simulink model "FIXED_BLOCK"  (R2024b)
settings: configuration reference "MODEL_CONFIG_CHILD" (kept outside this file)
undefined symbols (not defined in the file): BATTERY_UV_LIM_U16, BATTERY_UV_RST_LIM_U16, BOOLEAN_ONE, CONST_10000_u32, CONST_ONE_u8, CURR_CUTOFF_CTR_U16, CURRENTCUTOFF_LIM_mA_i32, DEFAULT_MAX_SPD_LIM_u16, DEFAULT_PAS_SPD_U16, DEFAULT_SPD_LIM_U16, ECO_MODE_SPD_LIM_u16, FITNESS_MODE_U8, MAX_SPD_VALUE_U16, MILLI_SEC_COUNTS_10000_U16, MILLI_SEC_COUNTS_1000_U16, MILLI_SEC_COUNTS_2000_U16, MILLI_SEC_COUNTS_3000_U16, MILLI_SEC_COUNTS_300_U16, MILLI_SEC_COUNTS_5000_U16, MIN_SPD_VALUE_U16, MOTOR_BLOCK_CTR_U16, PAS_FIVE_SPD_THSD_U16, PAS_FOUR_SPD_THSD_U16, PAS_ONE_SPD_THSD_U16, PAS_THREE_SPD_THSD_U16, PAS_TWO_SPD_THSD_U16, RPM_TO_KMPH_CONST_u32, SAMPLE_TIME_1MS, SPD_BUFFER_u16, SPD_CONV_METER_u16, SPD_PI_INIT_VAL_u16, SPD_PI_KI_u16, SPD_PI_KP_u16, THROTT_ERR_LWRTHSD_U16, THROTT_ERR_UPRTHSD_U16, THROTTLE_INITIATION_VALUE_U16, THROTTLE_SPD_LIM_U16, THROTTLE_THRESHOLD_U16, URBAN_MODE_SPD_LIM_u16, WALKMODE_SPD_LIM_U16, ZERO_i32, ZERO_U16
libraries: simulink x21, MCU_MAIN_LIB x7, slpidlib x1
settings Model: DataDictionary=MCU_FOC_MAIN_DD.sldd  EnableAccessToBaseWorkspace=off  Creator=415  LastModifiedBy=Shivaraj
settings ConfigSetRef: SourceName=MODEL_CONFIG_CHILD

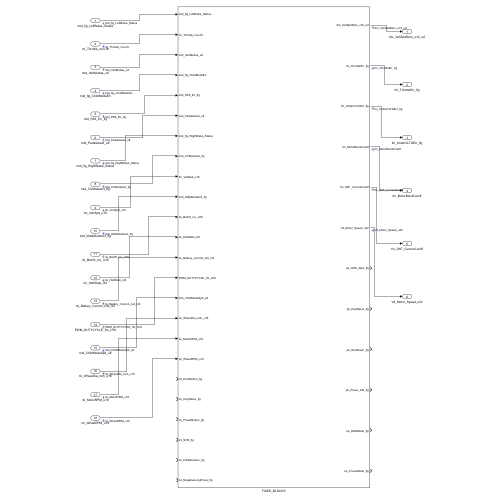
[thumbnail: Simulink's stored preview of the top-level diagram]
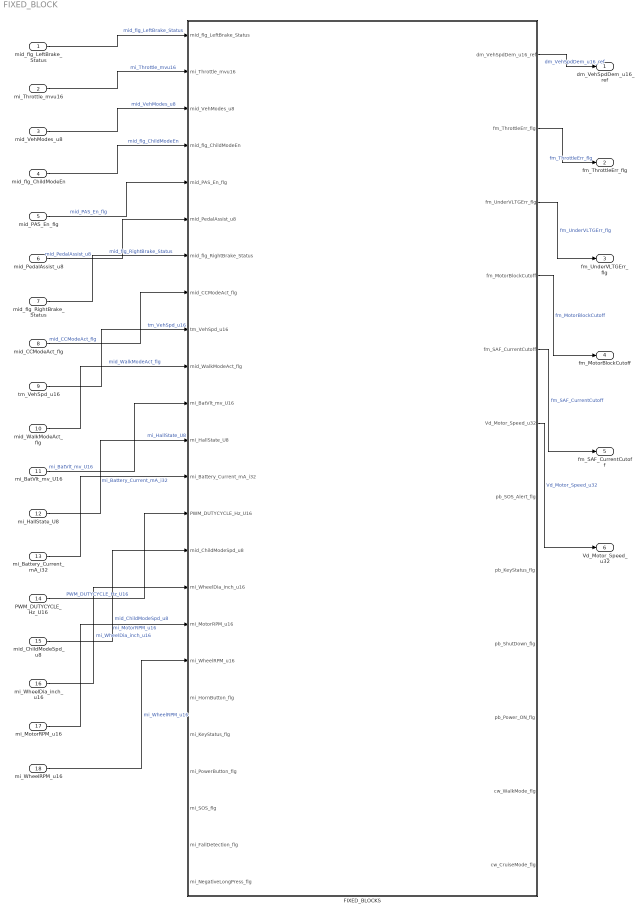
== system FIXED_BLOCK ==
  mid_flg_LeftBrake_Status : Inport
  mi_Throttle_mvu16 : Inport  Port=2
  mid_VehModes_u8 : Inport  Port=3
  mid_flg_ChildModeEn : Inport  Port=4
  mid_PAS_En_flg : Inport  Port=5
  mid_PedalAssist_u8 : Inport  Port=6
  mid_flg_RightBrake_Status : Inport  Port=7
  mid_CCModeAct_flg : Inport  Port=8
  tm_VehSpd_u16 : Inport  Port=9
  mid_WalkModeAct_flg : Inport  Port=10
  mi_BatVlt_mv_U16 : Inport  Port=11
  mi_HallState_U8 : Inport  Port=12
  mi_Battery_Current_mA_i32 : Inport  Port=13
  PWM_DUTYCYCLE_Hz_U16 : Inport  Port=14
  mid_ChildModeSpd_u8 : Inport  Port=15
  mi_WheelDia_inch_u16 : Inport  Port=16
  mi_MotorRPM_u16 : Inport  Port=17
  mi_WheelRPM_u16 : Inport  Port=18
  FIXED_BLOCKS : Subsystem
  dm_VehSpdDem_u16_ref : Outport  InitialOutput=0
  fm_ThrottleErr_flg : Outport  Port=2  InitialOutput=0
  fm_UnderVLTGErr_flg : Outport  Port=3  InitialOutput=0
  fm_MotorBlockCutoff : Outport  Port=4  InitialOutput=0
  fm_SAF_CurrentCutoff : Outport  Port=5
  Vd_Motor_Speed_u32 : Outport  Port=6  InitialOutput=0
  wires:
  FIXED_BLOCKS/4(fm_MotorBlockCutoff) -> fm_MotorBlockCutoff/1  "fm_MotorBlockCutoff"
  mid_flg_LeftBrake_Status/1 -> FIXED_BLOCKS/1(mid_flg_LeftBrake_Status)  "mid_flg_LeftBrake_Status"
  mi_Throttle_mvu16/1 -> FIXED_BLOCKS/2(mi_Throttle_mvu16)  "mi_Throttle_mvu16"
  tm_VehSpd_u16/1 -> FIXED_BLOCKS/9(tm_VehSpd_u16)  "tm_VehSpd_u16"
  mid_CCModeAct_flg/1 -> FIXED_BLOCKS/8(mid_CCModeAct_flg)  "mid_CCModeAct_flg"
  mid_ChildModeSpd_u8/1 -> FIXED_BLOCKS/15(mid_ChildModeSpd_u8)  "mid_ChildModeSpd_u8"
  mid_VehModes_u8/1 -> FIXED_BLOCKS/3(mid_VehModes_u8)  "mid_VehModes_u8"
  FIXED_BLOCKS/6(Vd_Motor_Speed_u32) -> Vd_Motor_Speed_u32/1  "Vd_Motor_Speed_u32"
  FIXED_BLOCKS/2(fm_ThrottleErr_flg) -> fm_ThrottleErr_flg/1  "fm_ThrottleErr_flg"
  mid_flg_ChildModeEn/1 -> FIXED_BLOCKS/4(mid_flg_ChildModeEn)  "mid_flg_ChildModeEn"
  mid_PAS_En_flg/1 -> FIXED_BLOCKS/5(mid_PAS_En_flg)  "mid_PAS_En_flg"
  mid_PedalAssist_u8/1 -> FIXED_BLOCKS/6(mid_PedalAssist_u8)  "mid_PedalAssist_u8"
  mid_flg_RightBrake_Status/1 -> FIXED_BLOCKS/7(mid_flg_RightBrake_Status)  "mid_flg_RightBrake_Status"
  mid_WalkModeAct_flg/1 -> FIXED_BLOCKS/10(mid_WalkModeAct_flg)  "mid_WalkModeAct_flg"
  mi_BatVlt_mv_U16/1 -> FIXED_BLOCKS/11(mi_BatVlt_mv_U16)  "mi_BatVlt_mv_U16"
  mi_HallState_U8/1 -> FIXED_BLOCKS/12(mi_HallState_U8)  "mi_HallState_U8"
  PWM_DUTYCYCLE_Hz_U16/1 -> FIXED_BLOCKS/14(PWM_DUTYCYCLE_Hz_U16)  "PWM_DUTYCYCLE_Hz_U16"
  mi_Battery_Current_mA_i32/1 -> FIXED_BLOCKS/13(mi_Battery_Current_mA_i32)  "mi_Battery_Current_mA_i32"
  mi_WheelDia_inch_u16/1 -> FIXED_BLOCKS/16(mi_WheelDia_inch_u16)  "mi_WheelDia_inch_u16"
  mi_MotorRPM_u16/1 -> FIXED_BLOCKS/17(mi_MotorRPM_u16)  "mi_MotorRPM_u16"
  mi_WheelRPM_u16/1 -> FIXED_BLOCKS/18(mi_WheelRPM_u16)  "mi_WheelRPM_u16"
  FIXED_BLOCKS/1(dm_VehSpdDem_u16_ref) -> dm_VehSpdDem_u16_ref/1  "dm_VehSpdDem_u16_ref"
  FIXED_BLOCKS/3(fm_UnderVLTGErr_flg) -> fm_UnderVLTGErr_flg/1  "fm_UnderVLTGErr_flg"
  FIXED_BLOCKS/5(fm_SAF_CurrentCutoff) -> fm_SAF_CurrentCutoff/1  "fm_SAF_CurrentCutoff"

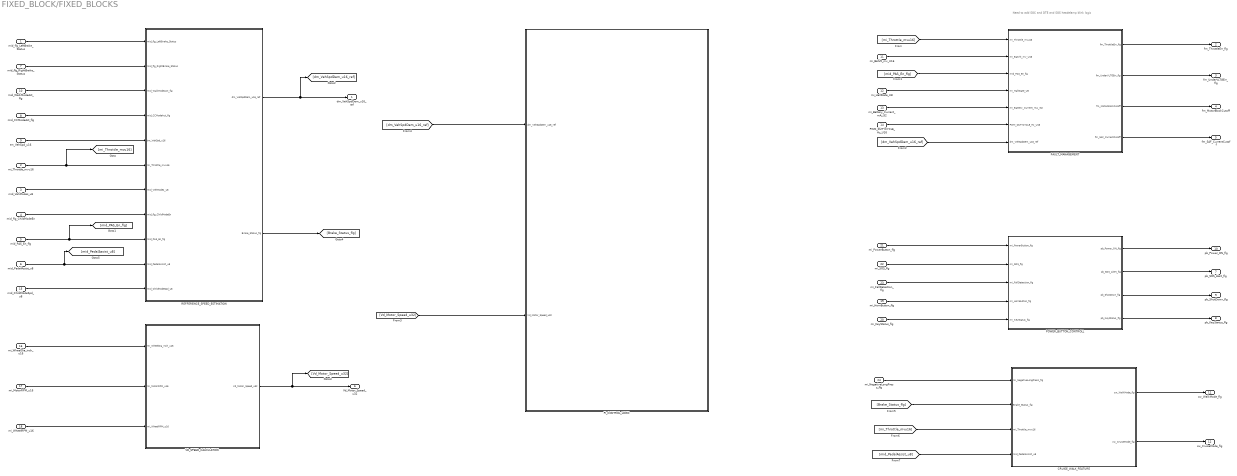
== system FIXED_BLOCK/FIXED_BLOCKS ==
  note: Need to add SOC and DTE and SOS headelamp blink logic
  mid_flg_LeftBrake_Status : Inport
  mi_Throttle_mvu16 : Inport  Port=2
  mid_VehModes_u8 : Inport  Port=3
  mid_flg_ChildModeEn : Inport  Port=4
  mid_PAS_En_flg : Inport  Port=5
  mid_PedalAssist_u8 : Inport  Port=6
  mid_flg_RightBrake_Status : Inport  Port=7
  mid_CCModeAct_flg : Inport  Port=8
  tm_VehSpd_u16 : Inport  Port=9
  mid_WalkModeAct_flg : Inport  Port=10
  mi_BatVlt_mv_U16 : Inport  Port=11
  mi_HallState_U8 : Inport  Port=12
  mi_Battery_Current_mA_i32 : Inport  Port=13
  PWM_DUTYCYCLE_Hz_U16 : Inport  Port=14
  mid_ChildModeSpd_u8 : Inport  Port=15
  mi_WheelDia_inch_u16 : Inport  Port=16
  mi_MotorRPM_u16 : Inport  Port=17
  mi_WheelRPM_u16 : Inport  Port=18
  mi_HornButton_flg : Inport  Port=19
  mi_KeyStatus_flg : Inport  Port=20
  mi_PowerButton_flg : Inport  Port=21
  mi_SOS_flg : Inport  Port=22
  mi_FallDetection_flg : Inport  Port=23
  mi_NegativeLongPress_flg : Inport  Port=24
  CRUISE_WALK_FEATURE : Subsystem
  FAULT_MANAGEMENT : Subsystem
  PI_CONTROL_LOGIC : Subsystem
  POWER_BUTTON_CONTROLL : Subsystem
  REFFERENCE_SPEED_ESTIMATION : Subsystem
  VD_SPEED_CALCULATION : Subsystem
  dm_VehSpdDem_u16_ref : Outport  InitialOutput=0
  fm_ThrottleErr_flg : Outport  Port=2
  fm_UnderVLTGErr_flg : Outport  Port=3
  fm_MotorBlockCutoff : Outport  Port=4
  fm_SAF_CurrentCutoff : Outport  Port=5
  Vd_Motor_Speed_u32 : Outport  Port=6  InitialOutput=0
  pb_SOS_Alert_flg : Outport  Port=7
  pb_KeyStatus_flg : Outport  Port=8
  pb_ShutDown_flg : Outport  Port=9
  pb_Power_ON_flg : Outport  Port=10
  cw_WalkMode_flg : Outport  Port=11
  cw_CruiseMode_flg : Outport  Port=12
  wires:
  mi_Throttle_mvu16/1 -> REFFERENCE_SPEED_ESTIMATION/6(mi_Throttle_mvu16), [mi_Throttle_mvu16]
  mid_flg_ChildModeEn/1 -> REFFERENCE_SPEED_ESTIMATION/8(mid_flg_ChildModeEn)
  mid_VehModes_u8/1 -> REFFERENCE_SPEED_ESTIMATION/7(mid_VehModes_u8)
  REFFERENCE_SPEED_ESTIMATION/1(dm_VehSpdDem_u16_ref) -> dm_VehSpdDem_u16_ref/1, [dm_VehSpdDem_u16_ref]
  mid_flg_RightBrake_Status/1 -> REFFERENCE_SPEED_ESTIMATION/2(mid_flg_RightBrake_Status)
  tm_VehSpd_u16/1 -> REFFERENCE_SPEED_ESTIMATION/5(tm_VehSpd_u16)
  mid_WalkModeAct_flg/1 -> REFFERENCE_SPEED_ESTIMATION/3(mid_WalkModeAct_flg)
  [mi_Throttle_mvu16] -> FAULT_MANAGEMENT/1(mi_Throttle_mvu16)
  mid_CCModeAct_flg/1 -> REFFERENCE_SPEED_ESTIMATION/4(mid_CCModeAct_flg)
  mid_PedalAssist_u8/1 -> [mid_PedalAssist_u8], REFFERENCE_SPEED_ESTIMATION/10(mid_PedalAssist_u8)
  mid_PAS_En_flg/1 -> [mid_PAS_En_flg], REFFERENCE_SPEED_ESTIMATION/9(mid_PAS_En_flg)
  mid_flg_LeftBrake_Status/1 -> REFFERENCE_SPEED_ESTIMATION/1(mid_flg_LeftBrake_Status)
  FAULT_MANAGEMENT/1(fm_ThrottleErr_flg) -> fm_ThrottleErr_flg/1
  mi_BatVlt_mv_U16/1 -> FAULT_MANAGEMENT/2(mi_BatVlt_mv_U16)
  [mid_PAS_En_flg] -> FAULT_MANAGEMENT/3(mid_PAS_En_flg)
  FAULT_MANAGEMENT/2(fm_UnderVLTGErr_flg) -> fm_UnderVLTGErr_flg/1
  FAULT_MANAGEMENT/3(fm_MotorBlockCutoff) -> fm_MotorBlockCutoff/1
  mi_HallState_U8/1 -> FAULT_MANAGEMENT/4(mi_HallState_U8)
  mi_Battery_Current_mA_i32/1 -> FAULT_MANAGEMENT/5(mi_Battery_Current_mA_i32)
  PWM_DUTYCYCLE_Hz_U16/1 -> FAULT_MANAGEMENT/6(PWM_DUTYCYCLE_Hz_U16)
  [dm_VehSpdDem_u16_ref] -> FAULT_MANAGEMENT/7(dm_VehSpdDem_u16_ref)
  FAULT_MANAGEMENT/4(fm_SAF_CurrentCutoff) -> fm_SAF_CurrentCutoff/1
  mid_ChildModeSpd_u8/1 -> REFFERENCE_SPEED_ESTIMATION/11(mid_ChildModeSpd_u8)
  mi_WheelDia_inch_u16/1 -> VD_SPEED_CALCULATION/1(mi_WheelDia_inch_u16)
  mi_MotorRPM_u16/1 -> VD_SPEED_CALCULATION/2(mi_MotorRPM_u16)
  mi_WheelRPM_u16/1 -> VD_SPEED_CALCULATION/3(mi_WheelRPM_u16)
  VD_SPEED_CALCULATION/1(Vd_Motor_Speed_u32) -> [Vd_Motor_Speed_u32], Vd_Motor_Speed_u32/1
  [dm_VehSpdDem_u16_ref] -> PI_CONTROL_LOGIC/1(dm_VehSpdDem_u16_ref)
  [Vd_Motor_Speed_u32] -> PI_CONTROL_LOGIC/2(Vd_Motor_Speed_u32)
  POWER_BUTTON_CONTROLL/2(pb_SOS_Alert_flg) -> pb_SOS_Alert_flg/1
  POWER_BUTTON_CONTROLL/4(pb_KeyStatus_flg) -> pb_KeyStatus_flg/1
  POWER_BUTTON_CONTROLL/3(pb_ShutDown_flg) -> pb_ShutDown_flg/1
  mi_HornButton_flg/1 -> POWER_BUTTON_CONTROLL/4(mi_HornButton_flg)
  mi_KeyStatus_flg/1 -> POWER_BUTTON_CONTROLL/5(mi_KeyStatus_flg)
  mi_FallDetection_flg/1 -> POWER_BUTTON_CONTROLL/3(mi_FallDetection_flg)
  mi_SOS_flg/1 -> POWER_BUTTON_CONTROLL/2(mi_SOS_flg)
  mi_PowerButton_flg/1 -> POWER_BUTTON_CONTROLL/1(mi_PowerButton_flg)
  POWER_BUTTON_CONTROLL/1(pb_Power_ON_flg) -> pb_Power_ON_flg/1
  REFFERENCE_SPEED_ESTIMATION/2(Brake_Status_flg) -> [Brake_Status_flg]
  [Brake_Status_flg] -> CRUISE_WALK_FEATURE/2(Brake_Status_flg)
  [mi_Throttle_mvu16] -> CRUISE_WALK_FEATURE/3(mi_Throttle_mvu16)
  [mid_PedalAssist_u8] -> CRUISE_WALK_FEATURE/4(mid_PedalAssist_u8)
  CRUISE_WALK_FEATURE/1(cw_WalkMode_flg) -> cw_WalkMode_flg/1
  CRUISE_WALK_FEATURE/2(cw_CruiseMode_flg) -> cw_CruiseMode_flg/1
  mi_NegativeLongPress_flg/1 -> CRUISE_WALK_FEATURE/1(mi_NegativeLongPress_flg)

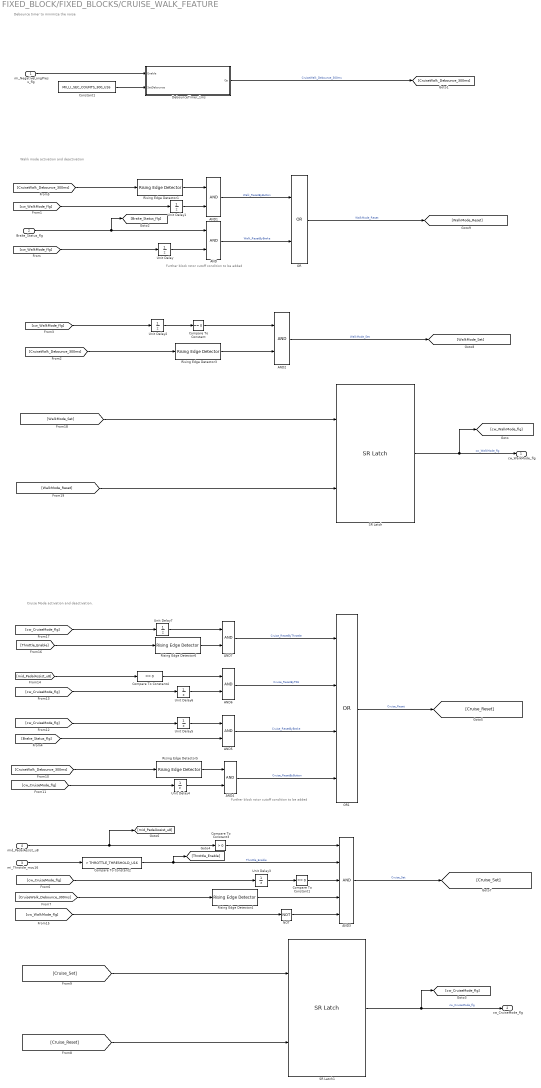
== system FIXED_BLOCK/FIXED_BLOCKS/CRUISE_WALK_FEATURE ==
  note: Debounce timer to minimize the noise
  note: Cruise Mode activation and deactivation.
  note: Walik mode activation and deactivation
  note: Further block rotor cutoff condition to be added
  note: Further block rotor cutoff condition to be added
  mi_NegativeLongPress_flg : Inport
  Brake_Status_flg : Inport  Port=2
  mi_Throttle_mvu16 : Inport  Port=3
  mid_PedalAssist_u8 : Inport  Port=4
  AND{,1..2,4..7} (7 alike) : Logic  AllPortsSameDT=off  OutDataTypeStr=boolean
  AND3 : Logic  Inputs=5  AllPortsSameDT=off  OutDataTypeStr=boolean
  Compare To Constant : simulink/Logic and Bit Operations/Compare To Constant  relop===  const=0  OutDataTypeStr=boolean
  Compare To Constant1 : simulink/Logic and Bit Operations/Compare To Constant  relop===  const=0  OutDataTypeStr=boolean
  Compare To Constant2 : simulink/Logic and Bit Operations/Compare To Constant  relop=>  const=THROTTLE_THRESHOLD_U16  OutDataTypeStr=boolean
  Compare To Constant3 : simulink/Logic and Bit Operations/Compare To Constant  relop=>  const=0  OutDataTypeStr=boolean
  Compare To Constant4 : simulink/Logic and Bit Operations/Compare To Constant  relop===  const=0  OutDataTypeStr=boolean
  Constant1 : Constant  Value=MILLI_SEC_COUNTS_300_U16
  DebounceTimer_1ms : Subsystem
  NOT : Logic  Operator=NOT  IconShape=distinctive  AllPortsSameDT=off  OutDataTypeStr=boolean
  OR : Logic  Operator=OR  AllPortsSameDT=off  OutDataTypeStr=boolean
  OR1 : Logic  Operator=OR  Inputs=4  AllPortsSameDT=off  OutDataTypeStr=boolean
  Rising Edge Detector{1,3..6} (5 alike) : MCU_MAIN_LIB/Rising Edge Detector  SystemSampleTime=-1  VariantActivationTime=update diagram  AllowFlexibleInterface=on  Latency=0  AutoFrameSizeCalculation=off
  SR Latch : MCU_MAIN_LIB/SR Latch  SystemSampleTime=-1  VariantActivationTime=update diagram  AllowFlexibleInterface=on  Latency=0  AutoFrameSizeCalculation=off
  SR Latch1 : MCU_MAIN_LIB/SR Latch  SystemSampleTime=-1  VariantActivationTime=update diagram  AllowFlexibleInterface=on  Latency=0  AutoFrameSizeCalculation=off
  Unit Delay{,1..7} (8 alike) : UnitDelay  SampleTime=-1  HasFrameUpgradeWarning=on
  cw_WalkMode_flg : Outport
  cw_CruiseMode_flg : Outport  Port=2
  wires:
  mi_NegativeLongPress_flg/1 -> DebounceTimer_1ms/1(Enable)
  Constant1/1 -> DebounceTimer_1ms/2(SetDebounce)
  SR Latch/1 -> [cw_WalkMode_flg], cw_WalkMode_flg/1  "cw_WalkMode_flg"
  AND/1 -> OR/2  "Walk_ResetByBrake"
  [cw_WalkMode_flg] -> Unit Delay/1
  Unit Delay/1 -> AND/2
  Brake_Status_flg/1 -> [Brake_Status_flg], AND/1
  Unit Delay1/1 -> AND1/2
  [cw_WalkMode_flg] -> Unit Delay1/1
  AND1/1 -> OR/1  "Walk_ResetByButton"
  Rising Edge Detector1/1 -> AND1/1
  [CruiseWalk_Debounce_300ms] -> Rising Edge Detector1/1
  DebounceTimer_1ms/1(Op) -> [CruiseWalk_Debounce_300ms]  "CruiseWalk_Debounce_300ms"
  [cw_WalkMode_flg] -> Unit Delay2/1
  Unit Delay2/1 -> Compare To Constant/1
  Compare To Constant/1 -> AND2/1
  SR Latch1/1 -> [cw_CruiseMode_flg], cw_CruiseMode_flg/1  "cw_CruiseMode_flg"
  Unit Delay3/1 -> Compare To Constant1/1
  [cw_CruiseMode_flg] -> Unit Delay3/1
  mi_Throttle_mvu16/1 -> Compare To Constant2/1
  Compare To Constant1/1 -> AND3/3
  [CruiseWalk_Debounce_300ms] -> Rising Edge Detector4/1
  Compare To Constant2/1 -> [Throttle_Enable], AND3/2  "Throttle_Enable"
  Compare To Constant3/1 -> AND3/1
  mid_PedalAssist_u8/1 -> [mid_PedalAssist_u8], Compare To Constant3/1
  Rising Edge Detector3/1 -> AND2/2
  Rising Edge Detector4/1 -> AND3/4
  [CruiseWalk_Debounce_300ms] -> Rising Edge Detector5/1
  Rising Edge Detector5/1 -> AND4/1
  [cw_CruiseMode_flg] -> Unit Delay4/1
  Unit Delay4/1 -> AND4/2
  Unit Delay5/1 -> AND5/1
  [cw_CruiseMode_flg] -> Unit Delay5/1
  Unit Delay6/1 -> AND6/2
  [cw_CruiseMode_flg] -> Unit Delay6/1
  [mid_PedalAssist_u8] -> Compare To Constant4/1
  Compare To Constant4/1 -> AND6/1
  [cw_WalkMode_flg] -> NOT/1
  NOT/1 -> AND3/5
  Rising Edge Detector6/1 -> AND7/2
  [Throttle_Enable] -> Rising Edge Detector6/1
  [cw_CruiseMode_flg] -> Unit Delay7/1
  Unit Delay7/1 -> AND7/1
  [CruiseWalk_Debounce_300ms] -> Rising Edge Detector3/1
  AND4/1 -> OR1/4  "Cruise_ResetByButton"
  [Brake_Status_flg] -> AND5/2
  AND7/1 -> OR1/1  "Cruise_ResetByThrottle"
  AND6/1 -> OR1/2  "Cruise_ResetByPAS"
  AND5/1 -> OR1/3  "Cruise_ResetByBrake"
  OR1/1 -> [Cruise_Reset]  "Cruise_Reset"
  [Cruise_Reset] -> SR Latch1/2
  AND3/1 -> [Cruise_Set]  "Cruise_Set"
  [Cruise_Set] -> SR Latch1/1
  AND2/1 -> [WalkMode_Set]  "WalkMode_Set"
  [WalkMode_Set] -> SR Latch/1
  OR/1 -> [WalkMode_Reset]  "WalkMode_Reset"
  [WalkMode_Reset] -> SR Latch/2

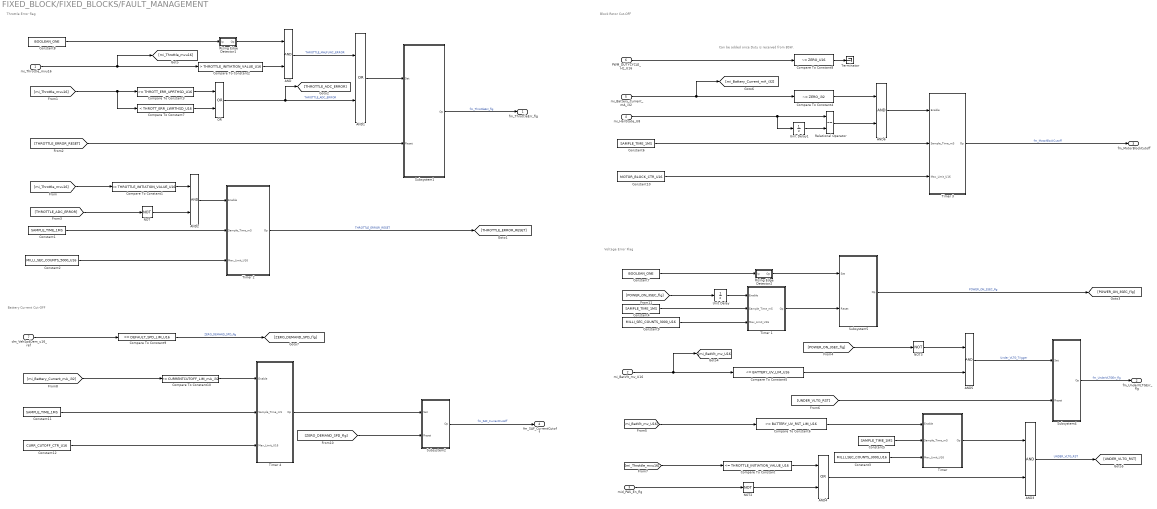
== system FIXED_BLOCK/FIXED_BLOCKS/FAULT_MANAGEMENT ==
  note: Battery Current Cut-OFF
  note: Can be added once Duty is received from BSW.
  note: Block Rotor Cut-OFF
  note: Voltage Error Flag
  note: Throttle Error flag
  mi_Throttle_mvu16 : Inport
  mi_BatVlt_mv_U16 : Inport  Port=2
  mid_PAS_En_flg : Inport  Port=3
  mi_HallState_U8 : Inport  Port=4
  mi_Battery_Current_mA_i32 : Inport  Port=5
  PWM_DUTYCYCLE_Hz_U16 : Inport  Port=6
  dm_VehSpdDem_u16_ref : Inport  Port=7
  AND{,2..3,5..6} (5 alike) : Logic  AllPortsSameDT=off  OutDataTypeStr=boolean
  AND1 : Logic  Operator=OR  AllPortsSameDT=off  OutDataTypeStr=boolean
  AND4 : Logic  Operator=OR  AllPortsSameDT=off  OutDataTypeStr=boolean
  Compare To Constant : simulink/Logic and Bit Operations/Compare To Constant  relop=<=  const=THROTTLE_INITIATION_VALUE_U16  OutDataTypeStr=boolean
  Compare To Constant1 : simulink/Logic and Bit Operations/Compare To Constant  relop=<=  const=THROTTLE_INITIATION_VALUE_U16  OutDataTypeStr=boolean
  Compare To Constant10 : simulink/Logic and Bit Operations/Compare To Constant  relop=>=  const=CURRENTCUTOFF_LIM_mA_i32  OutDataTypeStr=boolean
  Compare To Constant2 : simulink/Logic and Bit Operations/Compare To Constant  relop=>  const=THROTTLE_INITIATION_VALUE_U16  OutDataTypeStr=boolean
  Compare To Constant3 : simulink/Logic and Bit Operations/Compare To Constant  relop=>=  const=THROTT_ERR_UPRTHSD_U16  OutDataTypeStr=boolean
  Compare To Constant4 : simulink/Logic and Bit Operations/Compare To Constant  relop=~=  const=ZERO_i32  OutDataTypeStr=boolean
  Compare To Constant5 : simulink/Logic and Bit Operations/Compare To Constant  relop=<=  const=BATTERY_UV_LIM_U16  OutDataTypeStr=boolean
  Compare To Constant6 : simulink/Logic and Bit Operations/Compare To Constant  relop=>=  const=BATTERY_UV_RST_LIM_U16  OutDataTypeStr=boolean
  Compare To Constant7 : simulink/Logic and Bit Operations/Compare To Constant  relop=<  const=THROTT_ERR_LWRTHSD_U16  OutDataTypeStr=boolean
  Compare To Constant8 : simulink/Logic and Bit Operations/Compare To Constant  relop=~=  const=ZERO_U16  OutDataTypeStr=boolean
  Compare To Constant9 : simulink/Logic and Bit Operations/Compare To Constant  relop===  const=DEFAULT_SPD_LIM_U16  OutDataTypeStr=boolean
  Constant{1,4..6,11} (5 alike) : Constant  Value=SAMPLE_TIME_1MS
  Constant10 : Constant  Value=MOTOR_BLOCK_CTR_U16
  Constant12 : Constant  Value=CURR_CUTOFF_CTR_U16
  Constant2 : Constant  Value=MILLI_SEC_COUNTS_5000_U16
  Constant3 : Constant  Value=MILLI_SEC_COUNTS_3000_U16
  Constant7 : Constant  Value=BOOLEAN_ONE
  Constant8 : Constant  Value=BOOLEAN_ONE
  Constant9 : Constant  Value=MILLI_SEC_COUNTS_3000_U16
  NOT : Logic  Operator=NOT  IconShape=distinctive  AllPortsSameDT=off  OutDataTypeStr=boolean
  NOT2 : Logic  Operator=NOT  IconShape=distinctive  AllPortsSameDT=off  OutDataTypeStr=boolean
  NOT3 : Logic  Operator=NOT  IconShape=distinctive  AllPortsSameDT=off  OutDataTypeStr=boolean
  OR : Logic  Operator=OR  AllPortsSameDT=off  OutDataTypeStr=boolean
  Relational Operator : RelationalOperator  Operator===  OutDataTypeStr=boolean  RndMeth=Simplest  InputSameDT=off
  Rising Edge Detector1 : Subsystem
  Rising Edge Detector2 : Subsystem
  Subsystem1 : Subsystem
  Subsystem2 : Subsystem
  Subsystem4 : Subsystem
  Subsystem5 : Subsystem
  Terminator : Terminator
  "Timer " : Subsystem
  Timer 1 : Subsystem
  Timer 2 : Subsystem
  Timer 3 : Subsystem
  Timer 4 : Subsystem
  Unit Delay : UnitDelay  SampleTime=-1  HasFrameUpgradeWarning=on
  Unit Delay1 : UnitDelay  SampleTime=-1  HasFrameUpgradeWarning=on
  fm_ThrottleErr_flg : Outport
  fm_UnderVLTGErr_flg : Outport  Port=2
  fm_MotorBlockCutoff : Outport  Port=3  OutputWhenDisabled=reset  InitialOutput=0
  fm_SAF_CurrentCutoff : Outport  Port=4  OutputWhenDisabled=reset  InitialOutput=0
  wires:
  Constant8/1 -> Rising Edge Detector1/1(Ip)
  mi_Throttle_mvu16/1 -> Compare To Constant2/1, [mi_Throttle_mvu16]
  Compare To Constant2/1 -> AND/2
  Rising Edge Detector1/1(Op) -> AND/1
  AND/1 -> AND1/1  "THROTTLE_MALFUNC_ERROR"
  Timer 2/1(Op) -> [THROTTLE_ERROR_RESET]  "THROTTLE_ERROR_RESET"
  Constant1/1 -> Timer 2/2(Sample_Time_mS)
  Compare To Constant1/1 -> AND2/1
  [mi_Throttle_mvu16] -> Compare To Constant1/1
  Constant2/1 -> Timer 2/3(Max_Limit_U16)
  Subsystem1/1(Op) -> fm_ThrottleErr_flg/1  "fm_ThrottleErr_flg"
  Compare To Constant7/1 -> OR/2
  Compare To Constant3/1 -> OR/1
  [THROTTLE_ERROR_RESET] -> Subsystem1/2(Reset)
  AND1/1 -> Subsystem1/1(Set)
  [mi_Throttle_mvu16] -> Compare To Constant3/1, Compare To Constant7/1
  OR/1 -> [THROTTLE_ADC_ERROR], AND1/2  "THROTTLE_ADC_ERROR"
  [THROTTLE_ADC_ERROR] -> NOT/1
  NOT/1 -> AND2/2
  AND2/1 -> Timer 2/1(Enable)
  Unit Delay/1 -> Timer 1/1(Enable)
  NOT3/1 -> AND5/1
  NOT2/1 -> AND4/2
  Subsystem5/1(Op) -> [POWER_ON_3SEC_flg]  "POWER_ON_3SEC_flg"
  Subsystem4/1(Op) -> fm_UnderVLTGErr_flg/1  "fm_UnderVLTGErr_flg"
  Compare To Constant5/1 -> AND5/2
  mid_PAS_En_flg/1 -> NOT2/1
  [mi_Throttle_mvu16] -> Compare To Constant/1
  Constant9/1 -> Timer 1/3(Max_Limit_U16)
  Constant4/1 -> Timer 1/2(Sample_Time_mS)
  Constant5/1 -> "Timer "/2(Sample_Time_mS)
  Rising Edge Detector2/1(Op) -> Subsystem5/1(Set)
  Compare To Constant6/1 -> "Timer "/1(Enable)
  Compare To Constant/1 -> AND4/1
  [POWER_ON_3SEC_flg] -> Unit Delay/1
  Constant7/1 -> Rising Edge Detector2/1(Ip)
  AND5/1 -> Subsystem4/1(Set)  "Under_VLTG_Trigger"
  mi_BatVlt_mv_U16/1 -> [mi_BatVlt_mv_U16], Compare To Constant5/1
  "Timer "/1(Op) -> AND3/1
  AND4/1 -> AND3/2
  Timer 1/1(Op) -> Subsystem5/2(Reset)
  [UNDER_VLTG_RST] -> Subsystem4/2(Reset)
  Constant3/1 -> "Timer "/3(Max_Limit_U16)
  [POWER_ON_3SEC_flg] -> NOT3/1
  [mi_BatVlt_mv_U16] -> Compare To Constant6/1
  AND3/1 -> [UNDER_VLTG_RST]  "UNDER_VLTG_RST"
  Timer 3/1(Op) -> fm_MotorBlockCutoff/1  "fm_MotorBlockCutoff"
  AND6/1 -> Timer 3/1(Enable)
  Relational Operator/1 -> AND6/2
  Compare To Constant4/1 -> AND6/1
  mi_Battery_Current_mA_i32/1 -> Compare To Constant4/1, [mi_Battery_Current_mA_i32]
  Unit Delay1/1 -> Relational Operator/2
  mi_HallState_U8/1 -> Unit Delay1/1, Relational Operator/1
  Constant6/1 -> Timer 3/2(Sample_Time_mS)
  Constant10/1 -> Timer 3/3(Max_Limit_U16)
  Compare To Constant8/1 -> Terminator/1
  PWM_DUTYCYCLE_Hz_U16/1 -> Compare To Constant8/1
  Constant11/1 -> Timer 4/2(Sample_Time_mS)
  Compare To Constant10/1 -> Timer 4/1(Enable)
  [mi_Battery_Current_mA_i32] -> Compare To Constant10/1
  Timer 4/1(Op) -> Subsystem2/1(Set)
  Constant12/1 -> Timer 4/3(Max_Limit_U16)
  dm_VehSpdDem_u16_ref/1 -> Compare To Constant9/1
  Compare To Constant9/1 -> [ZERO_DEMAND_SPD_flg]  "ZERO_DEMAND_SPD_flg"
  [ZERO_DEMAND_SPD_flg] -> Subsystem2/2(Reset)
  Subsystem2/1(Op) -> fm_SAF_CurrentCutoff/1  "fm_SAF_CurrentCutoff"

== system FIXED_BLOCK/FIXED_BLOCKS/PI_CONTROL_LOGIC ==
  dm_VehSpdDem_u16_ref : Inport
  Vd_Motor_Speed_u32 : Inport  Port=2
  Add : Sum  Inputs=+-
  Constant : Constant  Value=SPD_PI_KP_u16
  Constant1 : Constant  Value=SPD_PI_KI_u16
  Constant2 : Constant  Value=SPD_PI_INIT_VAL_u16
  PID Controller : slpidlib/PID Controller  Controller=PI  Form=Parallel  TimeDomain=Discrete-time  UseExternalTs=off  SampleTime=-1  IntegratorMethod=Forward Euler  FilterMethod=Forward Euler  ControllerParametersSource=external  P=1  I=1  UseKiTs=on  D=0  UseExternalDerivativeSource=off  N=100  UseFilter=on  TunerSelectOption=Transfer Function Based (PID Tuner App)  InitialConditionSource=external  InitialConditionForIntegrator=0  InitialConditionForFilter=0  DifferentiatorICPrevScaledInput=0  ExternalReset=none  TrackingMode=off  Kt=1  LimitOutput=on  SatLimitsSource=external  UpperSaturationLimit=inf  LowerSaturationLimit=-inf  LinearizeAsGain=on  AntiWindupMode=none  Kb=1  LimitIntegrator=off  UpperIntegratorSaturationLimit=inf  LowerIntegratorSaturationLimit=-inf  SaturateOnIntegerOverflow=on  PGainOutDataTypeStr=Inherit: Inherit via back propagation  PProdOutDataTypeStr=Inherit: Inherit via back propagation  POutMin=[]  POutMax=[]  IGainOutDataTypeStr=Inherit: Inherit via back propagation  IProdOutDataTypeStr=Inherit: Inherit via back propagation  IOutMin=[]  IOutMax=[]  DOutMin=[]  DOutMax=[]  NOutMin=[]  NOutMax=[]  SumOutDataTypeStr=Inherit: Inherit via back propagation  SumOutMin=[]  SumOutMax=[]  SaturationOutMin=[]  SaturationOutMax=[]  PParamMin=[]  PParamMax=[]  IParamMin=[]  IParamMax=[]  DParamMin=[]  DParamMax=[]  NParamMin=[]  NParamMax=[]  KbParamMin=[]  KbParamMax=[]  KtParamMin=[]  KtParamMax=[]  KbOutMin=[]  KbOutMax=[]  KtOutMin=[]  KtOutMax=[]  IntegratorOutDataTypeStr=Inherit: Inherit via back propagation  IntegratorOutMin=[]  IntegratorOutMax=[]  FilterOutMin=[]  FilterOutMax=[]  SumI1OutMin=[]  SumI1OutMax=[]  SumI2OutMin=[]  SumI2OutMax=[]  SumI3OutMin=[]  SumI3OutMax=[]  SumI4OutMin=[]  SumI4OutMax=[]  SumDOutMin=[]  SumDOutMax=[]  DifferentiatorOutMin=[]  DifferentiatorOutMax=[]  FilterDiffOutCoefMin=[]  FilterDiffOutCoefMax=[]  ReciprocalOutMin=[]  ReciprocalOutMax=[]  SumDenOutMin=[]  SumDenOutMax=[]  SumNumOutMin=[]  SumNumOutMax=[]  DivideOutMin=[]  DivideOutMax=[]  UdiffTsProdOutMin=[]  UdiffTsProdOutMax=[]  NTsProdOutMin=[]  NTsProdOutMax=[]  UintegralTsProdOutMin=[]  UintegralTsProdOutMax=[]  UngainTsProdOutMin=[]  UngainTsProdOutMax=[]  ClampingZeroOutDataTypeStr=Inherit: Inherit via back propagation  ClampingZeroOutMin=[]  ClampingZeroOutMax=[]  FilterDenConstantOutDataTypeStr=Inherit: Inherit via back propagation  FilterDenConstantOutMin=[]  FilterDenConstantOutMax=[]  PCopyOutDataTypeStr=Inherit: Inherit via back propagation  PCopyOutMin=[]  PCopyOutMax=[]  NCopyOutDataTypeStr=Inherit: Inherit via back propagation  NCopyOutMin=[]  NCopyOutMax=[]  IntegratorContinuousStateAttributes=''  IntegratorStateMustResolveToSignalObject=off  IntegratorRTWStateStorageClass=Auto  FilterContinuousStateAttributes=''  FilterStateMustResolveToSignalObject=off  FilterRTWStateStorageClass=Auto  ParallelPVariant=ExternalParameters  IdealPVariant=Disabled  IVariant=ExternalParameters  DVariant=Disabled  IntegratorVariant=Discrete  SatVariant=External  AWVariant=Passthrough  PCopyVariant=Disabled  TRVariant=Disabled  FdbkBlocksVariant=Forward  IdealPFdbkVariant=Disabled  SatFdbkVariant=Disabled  DerivativeFilterVariant=Disabled  NVariant=Disabled  NCopyVariant=Disabled_SignalSpec  FilterICVariant=Disabled  IntegratorICVariant=ExternalICs  ExternalResetVariant=Disabled  TRSumVariant=Passthrough  SumFdbkVariant=Disabled  SumVariant=Sum_PI  TsampFilterVariant=InternalTs  TsampNgainVariant=Passthrough  TsampIntegralVariant=Disabled_SignalSpec  ExternalSaturationOutDataTypeStr=Inherit: Same as second input  DerivativeSourceVariant=Disabled  PreIntVariant=InternalPreInt
  wires:
  Constant2/1 -> PID Controller/4
  Constant1/1 -> PID Controller/3
  Constant/1 -> PID Controller/2
  Vd_Motor_Speed_u32/1 -> Add/2
  dm_VehSpdDem_u16_ref/1 -> Add/1
  Add/1 -> PID Controller/1

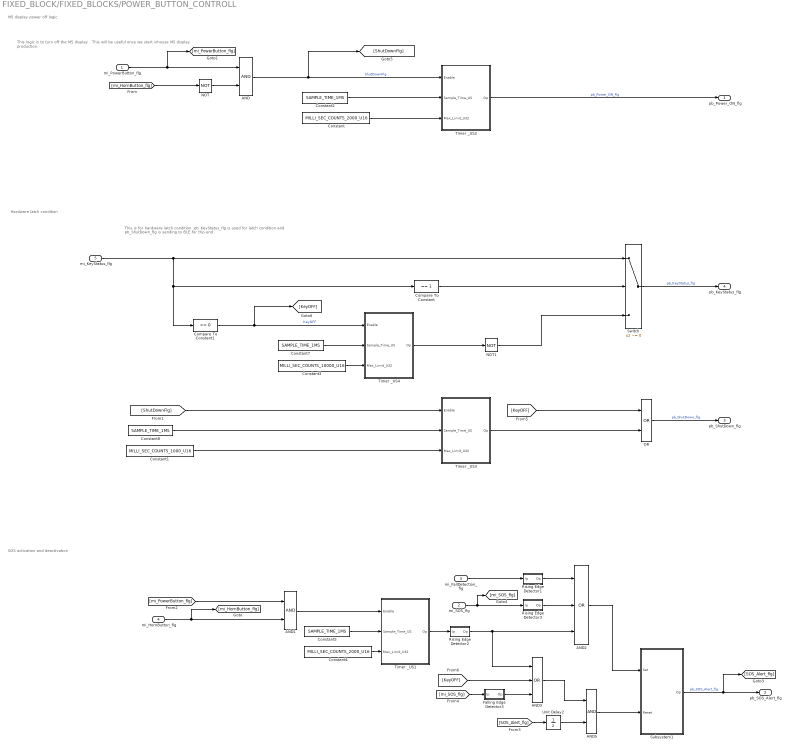
== system FIXED_BLOCK/FIXED_BLOCKS/POWER_BUTTON_CONTROLL ==
  note: This logic is to turn off the M5 display . This will be useful once we start inhouse M5 display production.
  note: M5 display power off logic
  note: This is for hardware latch condition .pb_KeyStatus_flg is used for latch condition and pb_ShutDown_flg is sending to BLE for trip end .
  note: Hardware latch condition
  note: SOS activation and deactivation
  mi_PowerButton_flg : Inport
  mi_SOS_flg : Inport  Port=2
  mi_FallDetection_flg : Inport  Port=3
  mi_HornButton_flg : Inport  Port=4
  mi_KeyStatus_flg : Inport  Port=5
  AND : Logic  AllPortsSameDT=off  OutDataTypeStr=boolean
  AND1 : Logic  AllPortsSameDT=off  OutDataTypeStr=boolean
  AND2 : Logic  Operator=OR  Inputs=3  AllPortsSameDT=off  OutDataTypeStr=boolean
  AND3 : Logic  Operator=OR  Inputs=3  AllPortsSameDT=off  OutDataTypeStr=boolean
  AND5 : Logic  AllPortsSameDT=off  OutDataTypeStr=boolean
  Compare To Constant : simulink/Logic and Bit Operations/Compare To Constant  relop===  const=1  OutDataTypeStr=boolean
  Compare To Constant1 : simulink/Logic and Bit Operations/Compare To Constant  relop===  const=0  OutDataTypeStr=boolean
  Constant : Constant  Value=MILLI_SEC_COUNTS_2000_U16
  Constant1 : Constant  Value=MILLI_SEC_COUNTS_1000_U16
  Constant{2,5,7..8} (4 alike) : Constant  Value=SAMPLE_TIME_1MS
  Constant3 : Constant  Value=MILLI_SEC_COUNTS_10000_U16
  Constant4 : Constant  Value=MILLI_SEC_COUNTS_2000_U16
  Falling Edge Detector3 : Subsystem
  NOT : Logic  Operator=NOT  AllPortsSameDT=off  OutDataTypeStr=boolean
  NOT1 : Logic  Operator=NOT  IconShape=distinctive  AllPortsSameDT=off  OutDataTypeStr=boolean
  OR : Logic  Operator=OR  AllPortsSameDT=off  OutDataTypeStr=boolean
  Rising Edge Detector1 : Subsystem
  Rising Edge Detector2 : Subsystem
  Rising Edge Detector3 : Subsystem
  Subsystem1 : Subsystem
  Switch : Switch  Criteria=u2 ~= 0  SaturateOnIntegerOverflow=off  InputSameDT=off
  Timer _US1 : Subsystem
  Timer _US2 : Subsystem
  Timer _US3 : Subsystem
  Timer _US4 : Subsystem
  Unit Delay2 : UnitDelay  SampleTime=-1  HasFrameUpgradeWarning=on
  pb_Power_ON_flg : Outport
  pb_SOS_Alert_flg : Outport  Port=2
  pb_ShutDown_flg : Outport  Port=3
  pb_KeyStatus_flg : Outport  Port=4
  wires:
  [KeyOFF] -> AND3/2
  OR/1 -> pb_ShutDown_flg/1  "pb_ShutDown_flg"
  [ShutDownFlg] -> Timer _US3/1(Enable)
  [KeyOFF] -> OR/1
  Compare To Constant/1 -> Switch/2
  Timer _US4/1(Op) -> NOT1/1
  NOT1/1 -> Switch/3
  Compare To Constant1/1 -> Timer _US4/1(Enable), [KeyOFF]  "KeyOFF"
  Switch/1 -> pb_KeyStatus_flg/1  "pb_KeyStatus_flg"
  mi_KeyStatus_flg/1 -> Compare To Constant/1, Compare To Constant1/1, Switch/1
  Constant7/1 -> Timer _US4/2(Sample_Time_US)
  Constant3/1 -> Timer _US4/3(Max_Limit_U32)
  Rising Edge Detector1/1(Op) -> AND2/1
  mi_FallDetection_flg/1 -> Rising Edge Detector1/1(Ip)
  Timer _US3/1(Op) -> OR/2
  Constant1/1 -> Timer _US3/3(Max_Limit_U32)
  Constant8/1 -> Timer _US3/2(Sample_Time_US)
  Unit Delay2/1 -> AND5/2
  [SOS_Alert_flg] -> Unit Delay2/1
  Rising Edge Detector3/1(Op) -> AND2/2
  [mi_SOS_flg] -> Falling Edge Detector3/1(Ip)
  AND5/1 -> Subsystem1/2(Reset)
  mi_SOS_flg/1 -> Rising Edge Detector3/1(Ip), [mi_SOS_flg]
  AND2/1 -> Subsystem1/1(Set)
  Rising Edge Detector2/1(Op) -> AND2/3, AND3/1
  AND1/1 -> Timer _US1/1(Enable)
  Constant5/1 -> Timer _US1/2(Sample_Time_US)
  Constant4/1 -> Timer _US1/3(Max_Limit_U32)
  Constant/1 -> Timer _US2/3(Max_Limit_U32)
  Constant2/1 -> Timer _US2/2(Sample_Time_US)
  AND/1 -> Timer _US2/1(Enable), [ShutDownFlg]  "ShutDownFlg"
  AND3/1 -> AND5/1
  Falling Edge Detector3/1(Op) -> AND3/3
  Subsystem1/1(Op) -> [SOS_Alert_flg], pb_SOS_Alert_flg/1  "pb_SOS_Alert_flg"
  Timer _US1/1(Op) -> Rising Edge Detector2/1(Ip)
  [mi_PowerButton_flg] -> AND1/1
  Timer _US2/1(Op) -> pb_Power_ON_flg/1  "pb_Power_ON_flg"
  NOT/1 -> AND/2
  [mi_HornButton_flg] -> NOT/1
  mi_HornButton_flg/1 -> [mi_HornButton_flg], AND1/2
  mi_PowerButton_flg/1 -> [mi_PowerButton_flg], AND/1

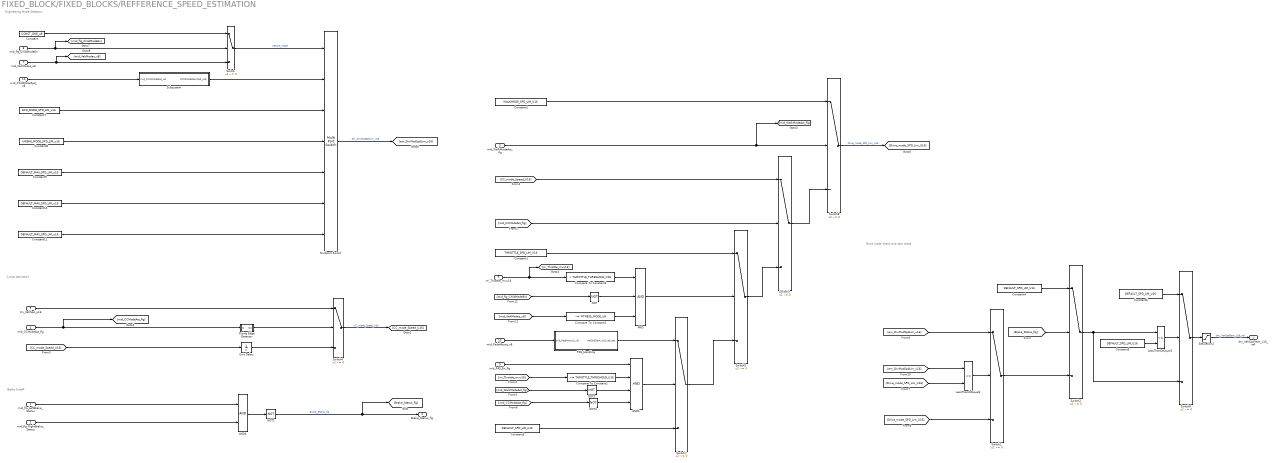
== system FIXED_BLOCK/FIXED_BLOCKS/REFFERENCE_SPEED_ESTIMATION ==
  note: Engineering Mode Selection
  note: Drive mode check and zero check
  note: Brake Cutoff
  note: Cruise Activation
  mid_flg_LeftBrake_Status : Inport
  mid_flg_RightBrake_Status : Inport  Port=2
  mid_WalkModeAct_flg : Inport  Port=3
  mid_CCModeAct_flg : Inport  Port=4
  tm_VehSpd_u16 : Inport  Port=5
  mi_Throttle_mvu16 : Inport  Port=6
  mid_VehModes_u8 : Inport  Port=7
  mid_flg_ChildModeEn : Inport  Port=8
  mid_PAS_En_flg : Inport  Port=9
  mid_PedalAssist_u8 : Inport  Port=10
  mid_ChildModeSpd_u8 : Inport  Port=11
  AND : Logic  Inputs=3  AllPortsSameDT=off  OutDataTypeStr=boolean
  AND1 : Logic  Inputs=4  AllPortsSameDT=off  OutDataTypeStr=boolean
  AND4 : Logic  AllPortsSameDT=off  OutDataTypeStr=boolean
  Compare To Constant1 : simulink/Logic and Bit Operations/Compare To Constant  relop=~=  const=FITNESS_MODE_U8  OutDataTypeStr=boolean
  Compare To Constant2 : simulink/Logic and Bit Operations/Compare To Constant  relop=<=  const=THROTTLE_THRESHOLD_U16  OutDataTypeStr=boolean
  Compare To Constant3 : simulink/Logic and Bit Operations/Compare To Constant  relop=>  const=THROTTLE_THRESHOLD_U16  OutDataTypeStr=boolean
  Constant : Constant  Value=CONST_ONE_u8
  Constant1 : Constant  Value=THROTTLE_SPD_LIM_U16
  Constant10 : Constant  Value=DEFAULT_MAX_SPD_LIM_u16
  Constant11 : Constant  Value=DEFAULT_MAX_SPD_LIM_u16
  Constant2 : Constant  Value=WALKMODE_SPD_LIM_U16
  Constant{3..6} (4 alike) : Constant  Value=DEFAULT_SPD_LIM_U16
  Constant7 : Constant  Value=ECO_MODE_SPD_LIM_u16
  Constant8 : Constant  Value=URBAN_MODE_SPD_LIM_u16
  Constant9 : Constant  Value=DEFAULT_MAX_SPD_LIM_u16
  LessThanOrEqual1 : RelationalOperator  Operator=<=  OutDataTypeStr=boolean  RndMeth=Simplest  InputSameDT=off
  LessThanOrEqual3 : RelationalOperator  Operator=<=  OutDataTypeStr=boolean  RndMeth=Simplest  InputSameDT=off
  Multiport Switch : MultiPortSwitch  DataPortOrder=Specify indices  DataPortIndices={1,2,3,4,5,6}  DiagnosticForDefault=Warning  SaturateOnIntegerOverflow=off  InputSameDT=off
  NOT{,1..3} (4 alike) : Logic  Operator=NOT  IconShape=distinctive  AllPortsSameDT=off  OutDataTypeStr=boolean
  PAS_Handling : Subsystem
  Rising Edge Detector : Subsystem
  Saturation2 : Saturate  UpperLimit=MAX_SPD_VALUE_U16  LowerLimit=MIN_SPD_VALUE_U16
  Subsystem : Subsystem
  Switch{,1..8} (9 alike) : Switch  Criteria=u2 ~= 0  SaturateOnIntegerOverflow=off  InputSameDT=off
  Unit Delay : UnitDelay  SampleTime=-1  HasFrameUpgradeWarning=on
  dm_VehSpdDem_u16_ref : Outport  InitialOutput=0
  Brake_Status_flg : Outport  Port=2
  wires:
  Saturation2/1 -> dm_VehSpdDem_u16_ref/1  "dm_VehSpdDem_u16_ref"
  Switch2/1 -> Switch6/3, LessThanOrEqual1/1
  Constant5/1 -> LessThanOrEqual1/2
  LessThanOrEqual1/1 -> Switch6/2
  Constant6/1 -> Switch6/1
  mid_flg_RightBrake_Status/1 -> AND4/2
  Constant4/1 -> Switch2/1
  Switch1/1 -> Switch2/3
  NOT1/1 -> Brake_Status_flg/1, [Brake_Status_flg]  "Brake_Status_flg"
  mid_flg_LeftBrake_Status/1 -> AND4/1
  AND4/1 -> NOT1/1
  Switch6/1 -> Saturation2/1
  [Brake_Status_flg] -> Switch2/2
  [em_DrvModSpdLim_u16] -> LessThanOrEqual3/1
  [Drive_mode_SPD_Lim_U16] -> LessThanOrEqual3/2
  mid_WalkModeAct_flg/1 -> [mid_WalkModeAct_flg], Switch8/2
  Constant2/1 -> Switch8/1
  Switch3/1 -> Switch8/3
  mid_CCModeAct_flg/1 -> [mid_CCModeAct_flg], Rising Edge Detector/1(Ip)
  tm_VehSpd_u16/1 -> Switch4/1
  Rising Edge Detector/1(Op) -> Switch4/2
  Switch4/1 -> [CC_mode_Speed_U16]  "CC_mode_Speed_U16"
  Unit Delay/1 -> Switch4/3
  [mid_CCModeAct_flg] -> Switch3/2
  [CC_mode_Speed_U16] -> Switch3/1
  [CC_mode_Speed_U16] -> Unit Delay/1
  Switch5/1 -> Switch3/3
  AND/1 -> Switch5/2
  Compare To Constant3/1 -> AND/1
  Compare To Constant1/1 -> AND/3
  mid_VehModes_u8/1 -> [mid_VehModes_u8], Switch/3
  Constant1/1 -> Switch5/1
  Switch7/1 -> Switch5/3
  PAS_Handling/1(VehSpdDem_u16_ref_pas) -> Switch7/1
  mid_PedalAssist_u8/1 -> PAS_Handling/1(mid_PedalAssist_u8)
  mid_PAS_En_flg/1 -> AND1/1
  Constant3/1 -> Switch7/3
  AND1/1 -> Switch7/2
  [mid_WalkModeAct_flg] -> NOT2/1
  [mid_CCModeAct_flg] -> NOT3/1
  NOT2/1 -> AND1/3
  NOT3/1 -> AND1/4
  Compare To Constant2/1 -> AND1/2
  [mi_Throttle_mvu16] -> Compare To Constant2/1
  LessThanOrEqual3/1 -> Switch1/2
  Switch8/1 -> [Drive_mode_SPD_Lim_U16]  "Drive_mode_SPD_Lim_U16"
  [em_DrvModSpdLim_u16] -> Switch1/1
  [Drive_mode_SPD_Lim_U16] -> Switch1/3
  NOT/1 -> AND/2
  mid_flg_ChildModeEn/1 -> [mid_flg_ChildModeEn], Switch/2
  Constant/1 -> Switch/1
  mi_Throttle_mvu16/1 -> [mi_Throttle_mvu16], Compare To Constant3/1
  [mid_flg_ChildModeEn] -> NOT/1
  [mid_VehModes_u8] -> Compare To Constant1/1
  Switch/1 -> Multiport Switch/1  "Vehicle_Mode"
  mid_ChildModeSpd_u8/1 -> Subsystem/1(mid_ChildModeSpd_u8)
  Subsystem/1(ChildModeDemSpd_u16) -> Multiport Switch/2
  Constant7/1 -> Multiport Switch/3
  Constant8/1 -> Multiport Switch/4
  Constant9/1 -> Multiport Switch/5
  Constant10/1 -> Multiport Switch/6
  Constant11/1 -> Multiport Switch/7
  Multiport Switch/1 -> [em_DrvModSpdLim_u16]  "em_DrvModSpdLim_u16"

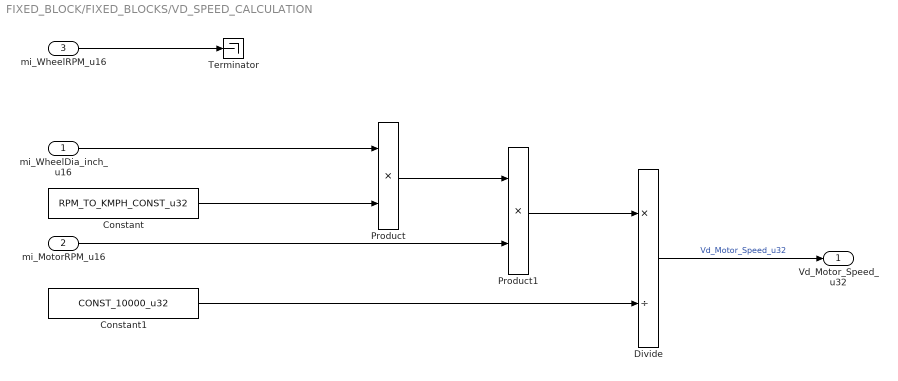
== system FIXED_BLOCK/FIXED_BLOCKS/VD_SPEED_CALCULATION ==
  mi_WheelDia_inch_u16 : Inport
  mi_MotorRPM_u16 : Inport  Port=2
  mi_WheelRPM_u16 : Inport  Port=3
  Constant : Constant  Value=RPM_TO_KMPH_CONST_u32
  Constant1 : Constant  Value=CONST_10000_u32
  Divide : Product  Inputs=*/  OutDataTypeStr=Inherit: Inherit via back propagation
  Product : Product  OutDataTypeStr=Inherit: Inherit via back propagation
  Product1 : Product  OutDataTypeStr=Inherit: Inherit via back propagation
  Terminator : Terminator
  Vd_Motor_Speed_u32 : Outport
  wires:
  Divide/1 -> Vd_Motor_Speed_u32/1  "Vd_Motor_Speed_u32"
  Constant1/1 -> Divide/2
  Product1/1 -> Divide/1
  mi_WheelRPM_u16/1 -> Terminator/1
  mi_MotorRPM_u16/1 -> Product1/2
  Product/1 -> Product1/1
  Constant/1 -> Product/2
  mi_WheelDia_inch_u16/1 -> Product/1

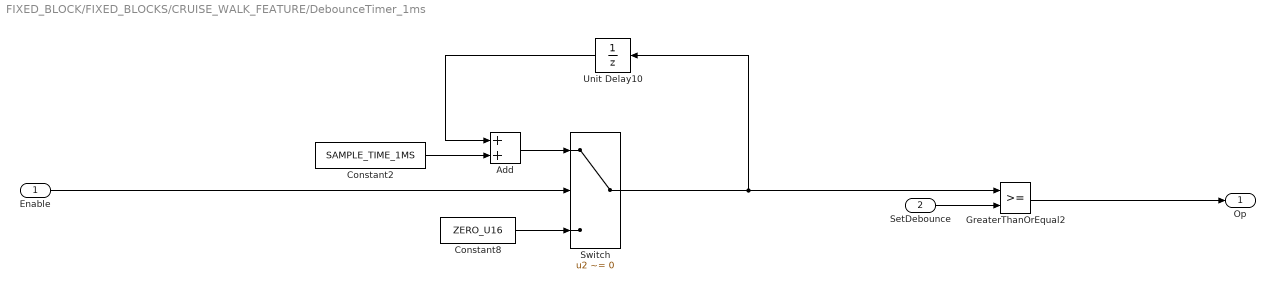
== system FIXED_BLOCK/FIXED_BLOCKS/CRUISE_WALK_FEATURE/DebounceTimer_1ms ==
  Enable : Inport
  SetDebounce : Inport  Port=2
  Add : Sum
  Constant2 : Constant  Value=SAMPLE_TIME_1MS
  Constant8 : Constant  Value=ZERO_U16
  GreaterThanOrEqual2 : RelationalOperator  OutDataTypeStr=boolean  RndMeth=Simplest  InputSameDT=off
  Switch : Switch  Criteria=u2 ~= 0  SaturateOnIntegerOverflow=off  InputSameDT=off
  Unit Delay10 : UnitDelay  SampleTime=-1  HasFrameUpgradeWarning=on
  Op : Outport
  wires:
  Constant2/1 -> Add/2
  Enable/1 -> Switch/2
  GreaterThanOrEqual2/1 -> Op/1
  SetDebounce/1 -> GreaterThanOrEqual2/2
  Constant8/1 -> Switch/3
  Unit Delay10/1 -> Add/1
  Switch/1 -> Unit Delay10/1, GreaterThanOrEqual2/1
  Add/1 -> Switch/1

== system FIXED_BLOCK/FIXED_BLOCKS/FAULT_MANAGEMENT/Rising Edge Detector1 ==
  Ip : Inport
  AND : Logic  AllPortsSameDT=off  OutDataTypeStr=boolean
  NOT : Logic  Operator=NOT  IconShape=distinctive  AllPortsSameDT=off  OutDataTypeStr=boolean
  Unit Delay : UnitDelay  SampleTime=-1  HasFrameUpgradeWarning=on
  Op : Outport
  wires:
  Unit Delay/1 -> NOT/1
  NOT/1 -> AND/2
  AND/1 -> Op/1
  Ip/1 -> AND/1, Unit Delay/1

== system FIXED_BLOCK/FIXED_BLOCKS/FAULT_MANAGEMENT/Rising Edge Detector2 ==
  Ip : Inport
  AND : Logic  AllPortsSameDT=off  OutDataTypeStr=boolean
  NOT : Logic  Operator=NOT  IconShape=distinctive  AllPortsSameDT=off  OutDataTypeStr=boolean
  Unit Delay : UnitDelay  SampleTime=-1  HasFrameUpgradeWarning=on
  Op : Outport
  wires:
  Ip/1 -> Unit Delay/1, AND/1
  AND/1 -> Op/1
  NOT/1 -> AND/2
  Unit Delay/1 -> NOT/1

== system FIXED_BLOCK/FIXED_BLOCKS/FAULT_MANAGEMENT/Subsystem1 ==
  Set : Inport
  Reset : Inport  Port=2
  AND : Logic  AllPortsSameDT=off  OutDataTypeStr=boolean
  AND1 : Logic  AllPortsSameDT=off  OutDataTypeStr=boolean
  NOT : Logic  Operator=NOT  IconShape=distinctive  AllPortsSameDT=off  OutDataTypeStr=boolean
  OR : Logic  Operator=OR  AllPortsSameDT=off  OutDataTypeStr=boolean
  Unit Delay : UnitDelay  SampleTime=-1  HasFrameUpgradeWarning=on
  Op : Outport
  wires:
  Reset/1 -> NOT/1
  OR/1 -> Unit Delay/1, Op/1
  NOT/1 -> AND1/1, AND/2
  Unit Delay/1 -> AND1/2
  Set/1 -> AND/1
  AND/1 -> OR/1
  AND1/1 -> OR/2

== system FIXED_BLOCK/FIXED_BLOCKS/FAULT_MANAGEMENT/Subsystem2 ==
  Set : Inport
  Reset : Inport  Port=2
  AND : Logic  AllPortsSameDT=off  OutDataTypeStr=boolean
  AND1 : Logic  AllPortsSameDT=off  OutDataTypeStr=boolean
  NOT : Logic  Operator=NOT  IconShape=distinctive  AllPortsSameDT=off  OutDataTypeStr=boolean
  OR : Logic  Operator=OR  AllPortsSameDT=off  OutDataTypeStr=boolean
  Unit Delay : UnitDelay  SampleTime=-1  HasFrameUpgradeWarning=on
  Op : Outport
  wires:
  AND1/1 -> OR/2
  AND/1 -> OR/1
  Set/1 -> AND/1
  Unit Delay/1 -> AND1/2
  NOT/1 -> AND/2, AND1/1
  OR/1 -> Op/1, Unit Delay/1
  Reset/1 -> NOT/1

== system FIXED_BLOCK/FIXED_BLOCKS/FAULT_MANAGEMENT/Subsystem4 ==
  Set : Inport
  Reset : Inport  Port=2
  AND : Logic  AllPortsSameDT=off  OutDataTypeStr=boolean
  AND1 : Logic  AllPortsSameDT=off  OutDataTypeStr=boolean
  NOT : Logic  Operator=NOT  IconShape=distinctive  AllPortsSameDT=off  OutDataTypeStr=boolean
  OR : Logic  Operator=OR  AllPortsSameDT=off  OutDataTypeStr=boolean
  Unit Delay : UnitDelay  SampleTime=-1  HasFrameUpgradeWarning=on
  Op : Outport
  wires:
  AND1/1 -> OR/2
  AND/1 -> OR/1
  Set/1 -> AND/1
  Unit Delay/1 -> AND1/2
  NOT/1 -> AND/2, AND1/1
  OR/1 -> Op/1, Unit Delay/1
  Reset/1 -> NOT/1

== system FIXED_BLOCK/FIXED_BLOCKS/FAULT_MANAGEMENT/Subsystem5 ==
  Set : Inport
  Reset : Inport  Port=2
  AND : Logic  AllPortsSameDT=off  OutDataTypeStr=boolean
  AND1 : Logic  AllPortsSameDT=off  OutDataTypeStr=boolean
  NOT : Logic  Operator=NOT  IconShape=distinctive  AllPortsSameDT=off  OutDataTypeStr=boolean
  OR : Logic  Operator=OR  AllPortsSameDT=off  OutDataTypeStr=boolean
  Unit Delay : UnitDelay  SampleTime=-1  HasFrameUpgradeWarning=on
  Op : Outport
  wires:
  Reset/1 -> NOT/1
  OR/1 -> Unit Delay/1, Op/1
  NOT/1 -> AND1/1, AND/2
  Unit Delay/1 -> AND1/2
  Set/1 -> AND/1
  AND/1 -> OR/1
  AND1/1 -> OR/2

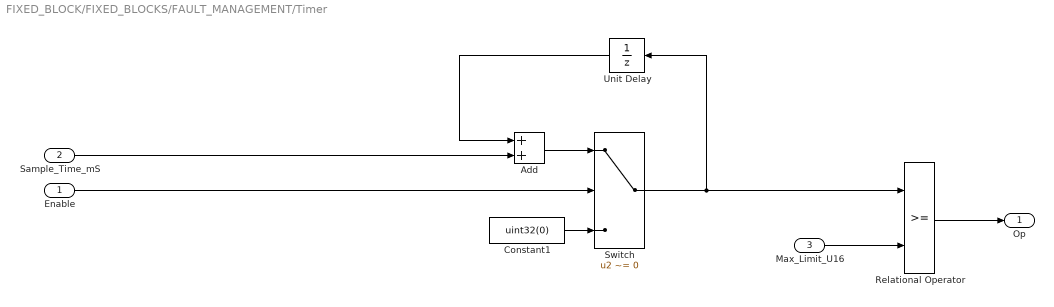
== system FIXED_BLOCK/FIXED_BLOCKS/FAULT_MANAGEMENT/Timer  ==
  Enable : Inport
  Sample_Time_mS : Inport  Port=2
  Max_Limit_U16 : Inport  Port=3
  Add : Sum
  Constant1 : Constant  Value=uint32(0)
  Relational Operator : RelationalOperator  OutDataTypeStr=boolean  RndMeth=Simplest  InputSameDT=off
  Switch : Switch  Criteria=u2 ~= 0  SaturateOnIntegerOverflow=off  InputSameDT=off
  Unit Delay : UnitDelay  SampleTime=-1  HasFrameUpgradeWarning=on
  Op : Outport
  wires:
  Max_Limit_U16/1 -> Relational Operator/2
  Relational Operator/1 -> Op/1
  Enable/1 -> Switch/2
  Constant1/1 -> Switch/3
  Add/1 -> Switch/1
  Sample_Time_mS/1 -> Add/2
  Unit Delay/1 -> Add/1
  Switch/1 -> Relational Operator/1, Unit Delay/1

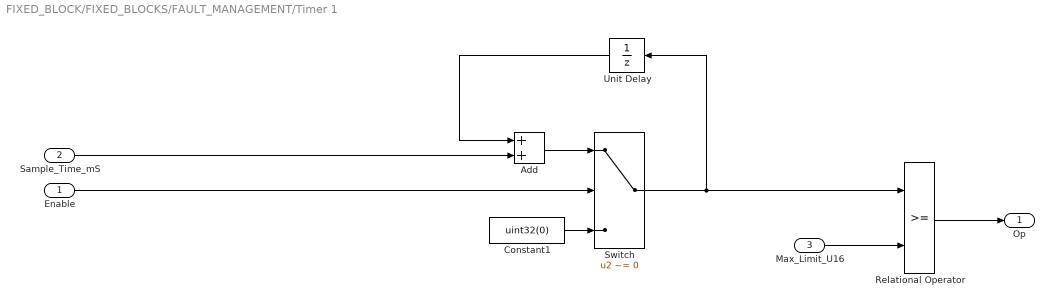
== system FIXED_BLOCK/FIXED_BLOCKS/FAULT_MANAGEMENT/Timer 1 ==
  Enable : Inport
  Sample_Time_mS : Inport  Port=2
  Max_Limit_U16 : Inport  Port=3
  Add : Sum
  Constant1 : Constant  Value=uint32(0)
  Relational Operator : RelationalOperator  OutDataTypeStr=boolean  RndMeth=Simplest  InputSameDT=off
  Switch : Switch  Criteria=u2 ~= 0  SaturateOnIntegerOverflow=off  InputSameDT=off
  Unit Delay : UnitDelay  SampleTime=-1  HasFrameUpgradeWarning=on
  Op : Outport
  wires:
  Switch/1 -> Unit Delay/1, Relational Operator/1
  Unit Delay/1 -> Add/1
  Sample_Time_mS/1 -> Add/2
  Add/1 -> Switch/1
  Constant1/1 -> Switch/3
  Enable/1 -> Switch/2
  Relational Operator/1 -> Op/1
  Max_Limit_U16/1 -> Relational Operator/2

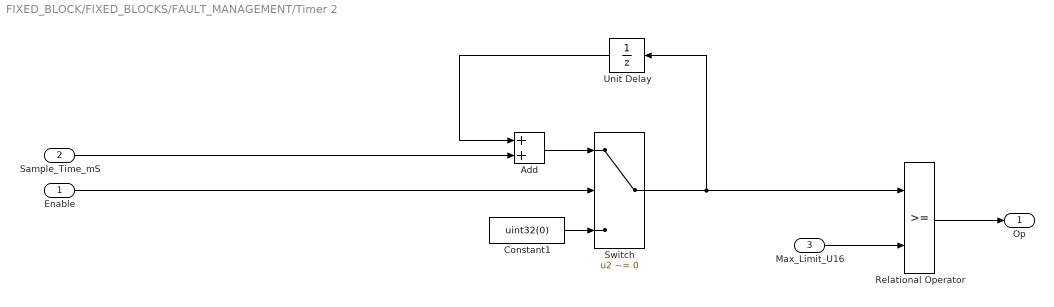
== system FIXED_BLOCK/FIXED_BLOCKS/FAULT_MANAGEMENT/Timer 2 ==
  Enable : Inport
  Sample_Time_mS : Inport  Port=2
  Max_Limit_U16 : Inport  Port=3
  Add : Sum
  Constant1 : Constant  Value=uint32(0)
  Relational Operator : RelationalOperator  OutDataTypeStr=boolean  RndMeth=Simplest  InputSameDT=off
  Switch : Switch  Criteria=u2 ~= 0  SaturateOnIntegerOverflow=off  InputSameDT=off
  Unit Delay : UnitDelay  SampleTime=-1  HasFrameUpgradeWarning=on
  Op : Outport
  wires:
  Max_Limit_U16/1 -> Relational Operator/2
  Relational Operator/1 -> Op/1
  Enable/1 -> Switch/2
  Constant1/1 -> Switch/3
  Add/1 -> Switch/1
  Sample_Time_mS/1 -> Add/2
  Unit Delay/1 -> Add/1
  Switch/1 -> Relational Operator/1, Unit Delay/1

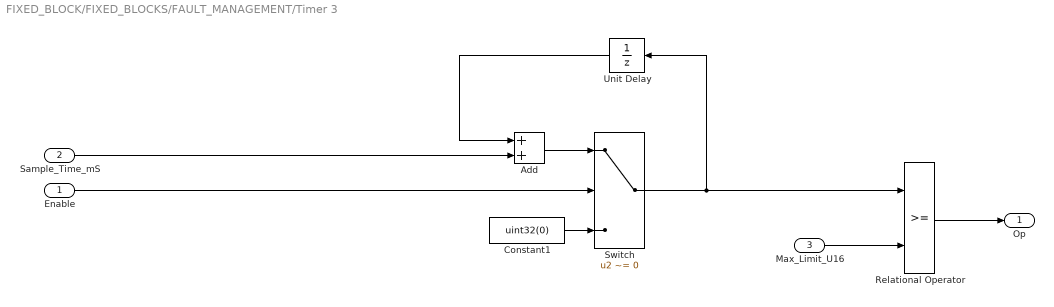
== system FIXED_BLOCK/FIXED_BLOCKS/FAULT_MANAGEMENT/Timer 3 ==
  Enable : Inport
  Sample_Time_mS : Inport  Port=2
  Max_Limit_U16 : Inport  Port=3
  Add : Sum
  Constant1 : Constant  Value=uint32(0)
  Relational Operator : RelationalOperator  OutDataTypeStr=boolean  RndMeth=Simplest  InputSameDT=off
  Switch : Switch  Criteria=u2 ~= 0  SaturateOnIntegerOverflow=off  InputSameDT=off
  Unit Delay : UnitDelay  SampleTime=-1  HasFrameUpgradeWarning=on
  Op : Outport
  wires:
  Switch/1 -> Unit Delay/1, Relational Operator/1
  Unit Delay/1 -> Add/1
  Sample_Time_mS/1 -> Add/2
  Add/1 -> Switch/1
  Constant1/1 -> Switch/3
  Enable/1 -> Switch/2
  Relational Operator/1 -> Op/1
  Max_Limit_U16/1 -> Relational Operator/2

== system FIXED_BLOCK/FIXED_BLOCKS/FAULT_MANAGEMENT/Timer 4 ==
  Enable : Inport
  Sample_Time_mS : Inport  Port=2
  Max_Limit_U16 : Inport  Port=3
  Add : Sum
  Constant1 : Constant  Value=uint32(0)
  Relational Operator : RelationalOperator  OutDataTypeStr=boolean  RndMeth=Simplest  InputSameDT=off
  Switch : Switch  Criteria=u2 ~= 0  SaturateOnIntegerOverflow=off  InputSameDT=off
  Unit Delay : UnitDelay  SampleTime=-1  HasFrameUpgradeWarning=on
  Op : Outport
  wires:
  Max_Limit_U16/1 -> Relational Operator/2
  Relational Operator/1 -> Op/1
  Enable/1 -> Switch/2
  Constant1/1 -> Switch/3
  Add/1 -> Switch/1
  Sample_Time_mS/1 -> Add/2
  Unit Delay/1 -> Add/1
  Switch/1 -> Relational Operator/1, Unit Delay/1

== system FIXED_BLOCK/FIXED_BLOCKS/POWER_BUTTON_CONTROLL/Falling Edge Detector3 ==
  Ip : Inport
  AND : Logic  AllPortsSameDT=off  OutDataTypeStr=boolean
  NOT1 : Logic  Operator=NOT  IconShape=distinctive  AllPortsSameDT=off  OutDataTypeStr=boolean
  Unit Delay : UnitDelay  SampleTime=-1  HasFrameUpgradeWarning=on
  Op : Outport
  wires:
  NOT1/1 -> AND/1
  Unit Delay/1 -> AND/2
  AND/1 -> Op/1
  Ip/1 -> NOT1/1, Unit Delay/1

== system FIXED_BLOCK/FIXED_BLOCKS/POWER_BUTTON_CONTROLL/Rising Edge Detector1 ==
  Ip : Inport
  AND : Logic  AllPortsSameDT=off  OutDataTypeStr=boolean
  NOT : Logic  Operator=NOT  IconShape=distinctive  AllPortsSameDT=off  OutDataTypeStr=boolean
  Unit Delay : UnitDelay  SampleTime=-1  HasFrameUpgradeWarning=on
  Op : Outport
  wires:
  Ip/1 -> Unit Delay/1, AND/1
  AND/1 -> Op/1
  NOT/1 -> AND/2
  Unit Delay/1 -> NOT/1

== system FIXED_BLOCK/FIXED_BLOCKS/POWER_BUTTON_CONTROLL/Rising Edge Detector2 ==
  Ip : Inport
  AND : Logic  AllPortsSameDT=off  OutDataTypeStr=boolean
  NOT : Logic  Operator=NOT  IconShape=distinctive  AllPortsSameDT=off  OutDataTypeStr=boolean
  Unit Delay : UnitDelay  SampleTime=-1  HasFrameUpgradeWarning=on
  Op : Outport
  wires:
  Ip/1 -> Unit Delay/1, AND/1
  AND/1 -> Op/1
  NOT/1 -> AND/2
  Unit Delay/1 -> NOT/1

== system FIXED_BLOCK/FIXED_BLOCKS/POWER_BUTTON_CONTROLL/Rising Edge Detector3 ==
  Ip : Inport
  AND : Logic  AllPortsSameDT=off  OutDataTypeStr=boolean
  NOT : Logic  Operator=NOT  IconShape=distinctive  AllPortsSameDT=off  OutDataTypeStr=boolean
  Unit Delay : UnitDelay  SampleTime=-1  HasFrameUpgradeWarning=on
  Op : Outport
  wires:
  Unit Delay/1 -> NOT/1
  NOT/1 -> AND/2
  AND/1 -> Op/1
  Ip/1 -> AND/1, Unit Delay/1

== system FIXED_BLOCK/FIXED_BLOCKS/POWER_BUTTON_CONTROLL/Subsystem1 ==
  Set : Inport
  Reset : Inport  Port=2
  AND : Logic  AllPortsSameDT=off  OutDataTypeStr=boolean
  AND1 : Logic  AllPortsSameDT=off  OutDataTypeStr=boolean
  NOT : Logic  Operator=NOT  IconShape=distinctive  AllPortsSameDT=off  OutDataTypeStr=boolean
  OR : Logic  Operator=OR  AllPortsSameDT=off  OutDataTypeStr=boolean
  Unit Delay : UnitDelay  SampleTime=-1  HasFrameUpgradeWarning=on
  Op : Outport
  wires:
  AND1/1 -> OR/2
  AND/1 -> OR/1
  Set/1 -> AND/1
  Unit Delay/1 -> AND1/2
  NOT/1 -> AND/2, AND1/1
  OR/1 -> Op/1, Unit Delay/1
  Reset/1 -> NOT/1

== system FIXED_BLOCK/FIXED_BLOCKS/POWER_BUTTON_CONTROLL/Timer _US1 ==
  Enable : Inport
  Sample_Time_US : Inport  Port=2
  Max_Limit_U32 : Inport  Port=3
  Add : Sum
  Constant1 : Constant  Value=uint32(0)
  Relational Operator : RelationalOperator  OutDataTypeStr=boolean  RndMeth=Simplest  InputSameDT=off
  Switch : Switch  Criteria=u2 ~= 0  SaturateOnIntegerOverflow=off  InputSameDT=off
  Unit Delay : UnitDelay  SampleTime=-1  HasFrameUpgradeWarning=on
  Op : Outport
  wires:
  Max_Limit_U32/1 -> Relational Operator/2
  Relational Operator/1 -> Op/1
  Enable/1 -> Switch/2
  Constant1/1 -> Switch/3
  Add/1 -> Switch/1
  Sample_Time_US/1 -> Add/2
  Unit Delay/1 -> Add/1
  Switch/1 -> Relational Operator/1, Unit Delay/1

== system FIXED_BLOCK/FIXED_BLOCKS/POWER_BUTTON_CONTROLL/Timer _US2 ==
  Enable : Inport
  Sample_Time_US : Inport  Port=2
  Max_Limit_U32 : Inport  Port=3
  Add : Sum
  Constant1 : Constant  Value=uint32(0)
  Relational Operator : RelationalOperator  OutDataTypeStr=boolean  RndMeth=Simplest  InputSameDT=off
  Switch : Switch  Criteria=u2 ~= 0  SaturateOnIntegerOverflow=off  InputSameDT=off
  Unit Delay : UnitDelay  SampleTime=-1  HasFrameUpgradeWarning=on
  Op : Outport
  wires:
  Switch/1 -> Unit Delay/1, Relational Operator/1
  Unit Delay/1 -> Add/1
  Sample_Time_US/1 -> Add/2
  Add/1 -> Switch/1
  Constant1/1 -> Switch/3
  Enable/1 -> Switch/2
  Relational Operator/1 -> Op/1
  Max_Limit_U32/1 -> Relational Operator/2

== system FIXED_BLOCK/FIXED_BLOCKS/POWER_BUTTON_CONTROLL/Timer _US3 ==
  Enable : Inport
  Sample_Time_US : Inport  Port=2
  Max_Limit_U32 : Inport  Port=3
  Add : Sum
  Constant1 : Constant  Value=uint32(0)
  Relational Operator : RelationalOperator  OutDataTypeStr=boolean  RndMeth=Simplest  InputSameDT=off
  Switch : Switch  Criteria=u2 ~= 0  SaturateOnIntegerOverflow=off  InputSameDT=off
  Unit Delay : UnitDelay  SampleTime=-1  HasFrameUpgradeWarning=on
  Op : Outport
  wires:
  Max_Limit_U32/1 -> Relational Operator/2
  Relational Operator/1 -> Op/1
  Enable/1 -> Switch/2
  Constant1/1 -> Switch/3
  Add/1 -> Switch/1
  Sample_Time_US/1 -> Add/2
  Unit Delay/1 -> Add/1
  Switch/1 -> Relational Operator/1, Unit Delay/1

== system FIXED_BLOCK/FIXED_BLOCKS/POWER_BUTTON_CONTROLL/Timer _US4 ==
  Enable : Inport
  Sample_Time_US : Inport  Port=2
  Max_Limit_U32 : Inport  Port=3
  Add : Sum
  Constant1 : Constant  Value=uint32(0)
  Relational Operator : RelationalOperator  OutDataTypeStr=boolean  RndMeth=Simplest  InputSameDT=off
  Switch : Switch  Criteria=u2 ~= 0  SaturateOnIntegerOverflow=off  InputSameDT=off
  Unit Delay : UnitDelay  SampleTime=-1  HasFrameUpgradeWarning=on
  Op : Outport
  wires:
  Switch/1 -> Unit Delay/1, Relational Operator/1
  Unit Delay/1 -> Add/1
  Sample_Time_US/1 -> Add/2
  Add/1 -> Switch/1
  Constant1/1 -> Switch/3
  Enable/1 -> Switch/2
  Relational Operator/1 -> Op/1
  Max_Limit_U32/1 -> Relational Operator/2

== system FIXED_BLOCK/FIXED_BLOCKS/REFFERENCE_SPEED_ESTIMATION/PAS_Handling ==
  mid_PedalAssist_u8 : Inport
  Constant : Constant  Value=PAS_ONE_SPD_THSD_U16
  Constant1 : Constant  Value=PAS_TWO_SPD_THSD_U16
  Constant2 : Constant  Value=PAS_THREE_SPD_THSD_U16
  Constant3 : Constant  Value=PAS_FOUR_SPD_THSD_U16
  Constant4 : Constant  Value=PAS_FIVE_SPD_THSD_U16
  Constant5 : Constant  Value=DEFAULT_PAS_SPD_U16
  Multiport Switch : MultiPortSwitch  DataPortOrder=Specify indices  DataPortIndices={1,2,3,4,5}  DataPortForDefault=Additional data port  DiagnosticForDefault=None  SaturateOnIntegerOverflow=off  InputSameDT=off
  VehSpdDem_u16_ref_pas : Outport
  wires:
  mid_PedalAssist_u8/1 -> Multiport Switch/1
  Constant/1 -> Multiport Switch/2
  Constant1/1 -> Multiport Switch/3
  Constant2/1 -> Multiport Switch/4
  Constant3/1 -> Multiport Switch/5
  Constant4/1 -> Multiport Switch/6
  Constant5/1 -> Multiport Switch/7
  Multiport Switch/1 -> VehSpdDem_u16_ref_pas/1

== system FIXED_BLOCK/FIXED_BLOCKS/REFFERENCE_SPEED_ESTIMATION/Rising Edge Detector ==
  Ip : Inport
  AND : Logic  AllPortsSameDT=off  OutDataTypeStr=boolean
  NOT : Logic  Operator=NOT  IconShape=distinctive  AllPortsSameDT=off  OutDataTypeStr=boolean
  Unit Delay : UnitDelay  SampleTime=-1  HasFrameUpgradeWarning=on
  Op : Outport
  wires:
  Ip/1 -> Unit Delay/1, AND/1
  AND/1 -> Op/1
  NOT/1 -> AND/2
  Unit Delay/1 -> NOT/1

== system FIXED_BLOCK/FIXED_BLOCKS/REFFERENCE_SPEED_ESTIMATION/Subsystem ==
  note: Check for data type coversion
  mid_ChildModeSpd_u8 : Inport
  Add : Sum
  Constant : Constant  Value=SPD_BUFFER_u16
  Constant1 : Constant  Value=SPD_CONV_METER_u16
  Product : Product
  ChildModeDemSpd_u16 : Outport
  wires:
  Constant/1 -> Add/2
  Product/1 -> Add/1
  Add/1 -> ChildModeDemSpd_u16/1  "ChildModeDemSpd_u16"
  Constant1/1 -> Product/2
  mid_ChildModeSpd_u8/1 -> Product/1
